simulink model "suspension_model"  (R2023b)
settings: Solver=VariableStepAuto  StartTime=0.0  StopTime=10.0  RelTol=1e-3
values from neighbouring files (symbols this model uses):
  C = 0    [LoadSuspensionParams.m]
  h_0 = 0    [LoadSuspensionParams.m]
  h_bump = 0.015    [LoadSuspensionParams.m]
  K = 5000    [LoadSuspensionParams.m]
  m = 12.5    [LoadSuspensionParams.m]
  T = 20    [LoadSuspensionParams.m]
  t_bump = w_bump/v    (= 1.2)    [LoadSuspensionParams.m]
libraries: simulink x1
settings Model: Creator=micha  LastModifiedBy=micha

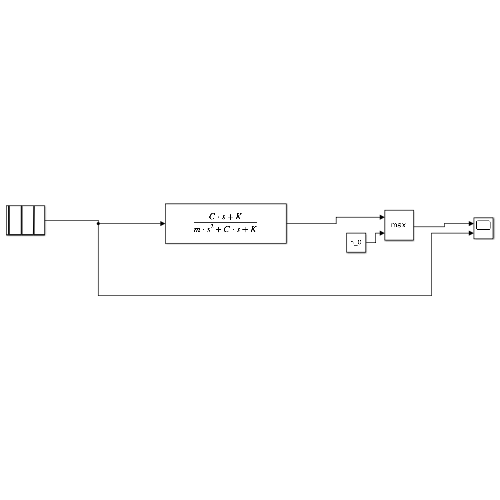
[thumbnail: Simulink's stored preview of the top-level diagram]
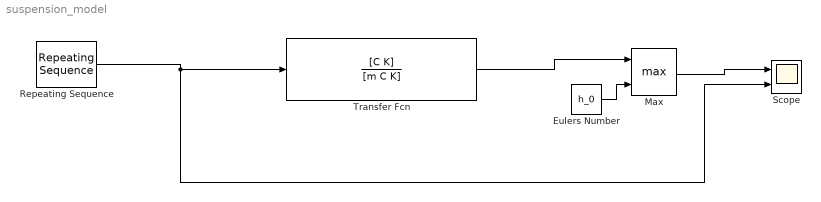
== system suspension_model ==
  Eulers Number : Constant  Value=h_0  OutDataTypeStr=Inherit: Inherit via back propagation
  Max : MinMax  Function=max  Inputs=2
  Repeating Sequence : simulink/Sources/Repeating Sequence  rep_seq_t="[0 2 2+t_bump*0.2  2+t_bump*0.8 2+t_bump T]"  rep_seq_y=[h_0 h_0 h_bump h_bump h_0 0]
  Scope : Scope  NumInputPorts=2
  Transfer Fcn : TransferFcn  Numerator=[C K]  Denominator=[m C K]
  wires:
  Repeating Sequence/1 -> Scope/2, Transfer Fcn/1
  Transfer Fcn/1 -> Max/1
  Max/1 -> Scope/1
  Eulers Number/1 -> Max/2
